simulink model "sampleModel7293_pp_1_1_mu"  (R2018a)
settings: Solver=VariableStepAuto  StartTime=0.0  StopTime=10.0  RelTol=1e-3
undefined symbols (not defined in the file): DiscIntNeverNeededParam
libraries: simulink x367
(part 10 of 13)

== system sampleModel7293_pp_1_1_mu/cfblk199/cfblk13 ==
  cfblk1 : Inport
  cfblk5 : Inport  Port=2
  cfblk6 : Inport  Port=3
  Action Port : ActionPort  ActionType=else
  cfblk3 : DiscreteFilter
  cfblk4 : simulink/Continuous/PID Controller  Controller=PID  TimeDomain=Discrete-time  SampleTime=-1  IntegratorMethod=Forward Euler  FilterMethod=Forward Euler  Form=Parallel  UseFilter=on  ControllerParametersSource=internal  P=1  I=1  D=0  N=100  InitialConditionSource=internal  InitialConditionForIntegrator=0  InitialConditionForFilter=0  ExternalReset=none  LimitOutput=off  UpperSaturationLimit=inf  LowerSaturationLimit=-inf  LinearizeAsGain=off  AntiWindupMode=none  Kb=1  TrackingMode=off  Kt=1  PParamMin=[]  PParamMax=[]  IParamMin=[]  IParamMax=[]  DParamMin=[]  DParamMax=[]  NParamMin=[]  NParamMax=[]  KbParamMin=[]  KbParamMax=[]  KtParamMin=[]  KtParamMax=[]  POutMin=[]  POutMax=[]  IOutMin=[]  IOutMax=[]  DOutMin=[]  DOutMax=[]  NOutMin=[]  NOutMax=[]  KbOutMin=[]  KbOutMax=[]  KtOutMin=[]  KtOutMax=[]  IntegratorOutMin=[]  IntegratorOutMax=[]  FilterOutMin=[]  FilterOutMax=[]  SumOutMin=[]  SumOutMax=[]  SumI1OutMin=[]  SumI1OutMax=[]  SumI2OutMin=[]  SumI2OutMax=[]  SumI3OutMin=[]  SumI3OutMax=[]  SumDOutMin=[]  SumDOutMax=[]  SaturationOutMin=[]  SaturationOutMax=[]  IntegratorContinuousStateAttributes=''  IntegratorStateMustResolveToSignalObject=off  IntegratorRTWStateStorageClass=Auto  FilterContinuousStateAttributes=''  FilterStateMustResolveToSignalObject=off  FilterRTWStateStorageClass=Auto  DifferentiatorICPrevScaledInput=0  DifferentiatorOutMin=[]  DifferentiatorOutMax=[]  FilterDiffOutCoefMin=[]  FilterDiffOutCoefMax=[]  SumDenOutMin=[]  SumDenOutMax=[]  SumNumOutMin=[]  SumNumOutMax=[]  ReciprocalOutMin=[]  ReciprocalOutMax=[]  DivideOutMin=[]  DivideOutMax=[]  TunerSelectOption=Transfer Function Based (PID Tuner App)
  cyemi_1105 : DataTypeConversion  OutDataTypeStr=double
  cyemi_1106 : DataTypeConversion  OutDataTypeStr=double
  cfblk2 : Outport
  cfblk7 : Outport  Port=2
  cfblk8 : Outport  Port=3
  cfblk9 : Outport  Port=4
  cfblk10 : Outport  Port=5
  wires:
  cfblk5/1 -> cfblk2/1, cfblk9/1
  cfblk6/1 -> cfblk10/1, cyemi_1106/1
  cfblk3/1 -> cfblk8/1
  cfblk4/1 -> cfblk7/1
  cyemi_1105/1 -> cfblk3/1
  cfblk1/1 -> cyemi_1105/1
  cyemi_1106/1 -> cfblk4/1

== system sampleModel7293_pp_1_1_mu/cfblk199/cfblk14 ==
  cfblk1 : Inport
  cfblk5 : Inport  Port=2
  cfblk6 : Inport  Port=3
  Action Port : ActionPort  ActionType=then
  cfblk3 : simulink/Discrete/Transfer Fcn First Order  PoleZ=0.95  ICPrevOutput=0.0  DoSatur=off
      settings: SourceProductName=Simulink
  cfblk4 : DiscreteZeroPole  Poles=[0 0.5]  Gain=1  SampleTime=-1
  cyemi_1110 : DataTypeConversion  OutDataTypeStr=double
  cyemi_1111 : DataTypeConversion  OutDataTypeStr=double
  cfblk2 : Outport
  cfblk7 : Outport  Port=2
  wires:
  cfblk6/1 -> cfblk7/1
  cfblk3/1 -> cfblk2/1
  cyemi_1110/1 -> cfblk3/1
  cfblk1/1 -> cyemi_1110/1
  cyemi_1111/1 -> cfblk4/1
  cfblk5/1 -> cyemi_1111/1

== system sampleModel7293_pp_1_1_mu/cfblk199/cfblk15 ==
  cfblk1 : Inport
  cfblk9 : Inport  Port=2
  cfblk10 : Inport  Port=3
  cfblk11 : Inport  Port=4
  Action Port : ActionPort  ActionType=else
  cfblk3 : DiscreteIntegrator  SampleTime=-1  OutDataTypeStr=double  ICPrevOutput=DiscIntNeverNeededParam  ICPrevScaledInput=DiscIntNeverNeededParam
  cfblk4 : simulink/Continuous/PID Controller (2DOF)  Controller=PID  TimeDomain=Discrete-time  SampleTime=-1  IntegratorMethod=Forward Euler  FilterMethod=Forward Euler  Form=Parallel  UseFilter=on  ControllerParametersSource=internal  P=1  I=1  D=0  N=100  b=1  c=1  InitialConditionSource=internal  InitialConditionForIntegrator=0  InitialConditionForFilter=0  ExternalReset=none  LimitOutput=off  UpperSaturationLimit=inf  LowerSaturationLimit=-inf  LinearizeAsGain=off  AntiWindupMode=none  Kb=1  TrackingMode=off  Kt=1  PParamMin=[]  PParamMax=[]  IParamMin=[]  IParamMax=[]  DParamMin=[]  DParamMax=[]  NParamMin=[]  NParamMax=[]  bParamMin=[]  bParamMax=[]  cParamMin=[]  cParamMax=[]  KbParamMin=[]  KbParamMax=[]  KtParamMin=[]  KtParamMax=[]  POutMin=[]  POutMax=[]  IOutMin=[]  IOutMax=[]  DOutMin=[]  DOutMax=[]  NOutMin=[]  NOutMax=[]  bOutMin=[]  bOutMax=[]  cOutMin=[]  cOutMax=[]  KbOutMin=[]  KbOutMax=[]  KtOutMin=[]  KtOutMax=[]  IntegratorOutMin=[]  IntegratorOutMax=[]  FilterOutMin=[]  FilterOutMax=[]  SumOutMin=[]  SumOutMax=[]  Sum1OutMin=[]  Sum1OutMax=[]  Sum2OutMin=[]  Sum2OutMax=[]  Sum3OutMin=[]  Sum3OutMax=[]  SumI1OutMin=[]  SumI1OutMax=[]  SumI2OutMin=[]  SumI2OutMax=[]  SumI3OutMin=[]  SumI3OutMax=[]  SumDOutMin=[]  SumDOutMax=[]  SaturationOutMin=[]  SaturationOutMax=[]  IntegratorContinuousStateAttributes=''  IntegratorStateMustResolveToSignalObject=off  IntegratorRTWStateStorageClass=Auto  FilterContinuousStateAttributes=''  FilterStateMustResolveToSignalObject=off  FilterRTWStateStorageClass=Auto  DifferentiatorICPrevScaledInput=0  DifferentiatorOutMin=[]  DifferentiatorOutMax=[]  FilterDiffOutCoefMin=[]  FilterDiffOutCoefMax=[]  SumDenOutMin=[]  SumDenOutMax=[]  SumNumOutMin=[]  SumNumOutMax=[]  ReciprocalOutMin=[]  ReciprocalOutMax=[]  DivideOutMin=[]  DivideOutMax=[]  TunerSelectOption=Transfer Function Based (PID Tuner App)
  cfblk5 : simulink/Discrete/Transfer Fcn Real Zero  ZeroZ=0.75  ICPrevInput=0.0  DoSatur=off
      settings: SourceProductName=Simulink  SourceProductBaseCode=SL
  cfblk6 : DiscreteFilter
  cfblk7 : simulink/Continuous/PID Controller  Controller=PID  TimeDomain=Discrete-time  SampleTime=-1  IntegratorMethod=Forward Euler  FilterMethod=Forward Euler  Form=Parallel  UseFilter=on  ControllerParametersSource=internal  P=1  I=1  D=0  N=100  InitialConditionSource=internal  InitialConditionForIntegrator=0  InitialConditionForFilter=0  ExternalReset=none  LimitOutput=off  UpperSaturationLimit=inf  LowerSaturationLimit=-inf  LinearizeAsGain=off  AntiWindupMode=none  Kb=1  TrackingMode=off  Kt=1  PParamMin=[]  PParamMax=[]  IParamMin=[]  IParamMax=[]  DParamMin=[]  DParamMax=[]  NParamMin=[]  NParamMax=[]  KbParamMin=[]  KbParamMax=[]  KtParamMin=[]  KtParamMax=[]  POutMin=[]  POutMax=[]  IOutMin=[]  IOutMax=[]  DOutMin=[]  DOutMax=[]  NOutMin=[]  NOutMax=[]  KbOutMin=[]  KbOutMax=[]  KtOutMin=[]  KtOutMax=[]  IntegratorOutMin=[]  IntegratorOutMax=[]  FilterOutMin=[]  FilterOutMax=[]  SumOutMin=[]  SumOutMax=[]  SumI1OutMin=[]  SumI1OutMax=[]  SumI2OutMin=[]  SumI2OutMax=[]  SumI3OutMin=[]  SumI3OutMax=[]  SumDOutMin=[]  SumDOutMax=[]  SaturationOutMin=[]  SaturationOutMax=[]  IntegratorContinuousStateAttributes=''  IntegratorStateMustResolveToSignalObject=off  IntegratorRTWStateStorageClass=Auto  FilterContinuousStateAttributes=''  FilterStateMustResolveToSignalObject=off  FilterRTWStateStorageClass=Auto  DifferentiatorICPrevScaledInput=0  DifferentiatorOutMin=[]  DifferentiatorOutMax=[]  FilterDiffOutCoefMin=[]  FilterDiffOutCoefMax=[]  SumDenOutMin=[]  SumDenOutMax=[]  SumNumOutMin=[]  SumNumOutMax=[]  ReciprocalOutMin=[]  ReciprocalOutMax=[]  DivideOutMin=[]  DivideOutMax=[]  TunerSelectOption=Transfer Function Based (PID Tuner App)
  cfblk8 : simulink/Discrete/Difference  ICPrevInput=0.0  OutMin=[]  OutMax=[]  OutDataTypeStr=double  OutputDataTypeScalingMode=double  OutDataType=fixdt(1, 16)  OutScaling=2^-10  DoSatur=off
  cyemi_{1116..1122} (7 alike) : DataTypeConversion  OutDataTypeStr=double
  cfblk2 : Outport
  cfblk12 : Outport  Port=2
  cfblk13 : Outport  Port=3
  cfblk14 : Outport  Port=4
  wires:
  cfblk4/1 -> cfblk12/1
  cfblk11/1 -> cyemi_1117/1, cyemi_1120/1
  cfblk8/1 -> cfblk14/1
  cfblk6/1 -> cfblk2/1
  cfblk1/1 -> cfblk13/1
  cyemi_1116/1 -> cfblk3/1
  cfblk7/1 -> cyemi_1116/1
  cyemi_1117/1 -> cfblk4/1
  cyemi_1118/1 -> cfblk4/2
  cfblk10/1 -> cyemi_1118/1
  cyemi_1119/1 -> cfblk5/1
  cfblk9/1 -> cyemi_1119/1
  cyemi_1120/1 -> cfblk6/1
  cyemi_1121/1 -> cfblk7/1
  cfblk5/1 -> cyemi_1121/1
  cyemi_1122/1 -> cfblk8/1
  cfblk3/1 -> cyemi_1122/1

== system sampleModel7293_pp_1_1_mu/cfblk199/cfblk22 ==
  emi_1180 : Inport
  Action Port : ActionPort  ActionType=then
  cfblk22 : Delay
  emi_1181 : Outport
  wires:
  emi_1180/1 -> cfblk22/1
  cfblk22/1 -> emi_1181/1

== system sampleModel7293_pp_1_1_mu/cfblk199/cfblk24 ==
  emi_1807 : Inport
  Action Port : ActionPort  ActionType=then
  cfblk24 : Delay
  emi_1808 : Outport
  wires:
  emi_1807/1 -> cfblk24/1
  cfblk24/1 -> emi_1808/1

== system sampleModel7293_pp_1_1_mu/cfblk199/cfblk5 ==
  emi_1529 : Inport
  Action Port : ActionPort  ActionType=then
  cfblk5 : DiscreteFir
  emi_1530 : Outport
  wires:
  emi_1529/1 -> cfblk5/1
  cfblk5/1 -> emi_1530/1

== system sampleModel7293_pp_1_1_mu/cfblk199/cfblk7 ==
  emi_832 : Inport
  Action Port : ActionPort  ActionType=then
  cfblk7 : UnitDelay  SampleTime=-1
  emi_833 : Outport
  wires:
  emi_832/1 -> cfblk7/1
  cfblk7/1 -> emi_833/1

== system sampleModel7293_pp_1_1_mu/cfblk199/emi_1182 ==
  Action Port : ActionPort  ActionType=else
  emi_1183 : Assertion

== system sampleModel7293_pp_1_1_mu/cfblk199/emi_1531 ==
  Action Port : ActionPort  ActionType=else
  emi_1532 : Assertion

== system sampleModel7293_pp_1_1_mu/cfblk199/emi_1809 ==
  Action Port : ActionPort  ActionType=else
  emi_1810 : Assertion

== system sampleModel7293_pp_1_1_mu/cfblk199/emi_834 ==
  Action Port : ActionPort  ActionType=else
  emi_835 : Assertion

== system sampleModel7293_pp_1_1_mu/cfblk200/cfblk11 ==
  cfblk1 : Inport
  Action Port : ActionPort  ActionType=then
  cfblk10 : simulink/Discrete/Transfer Fcn Lead or Lag  PoleZ=0.95  ZeroZ=0.75  ICPrevOutput=0.0  ICPrevInput=0.0  DoSatur=off
      settings: SourceProductName=Simulink  SourceProductBaseCode=SL
  cfblk11 : simulink/Discrete/Tapped Delay  vinit=0.0  samptime=-1  NumDelays=1  DelayOrder=Oldest  includeCurrent=off
  cfblk12 : Delay
  cfblk3 : Subsystem  TreatAsAtomicUnit=on
  cfblk4 : DiscreteTransferFcn
  cfblk5 : simulink/Continuous/PID Controller  Controller=PID  TimeDomain=Discrete-time  SampleTime=-1  IntegratorMethod=Forward Euler  FilterMethod=Forward Euler  Form=Parallel  UseFilter=on  ControllerParametersSource=internal  P=1  I=1  D=0  N=100  InitialConditionSource=internal  InitialConditionForIntegrator=0  InitialConditionForFilter=0  ExternalReset=none  LimitOutput=off  UpperSaturationLimit=inf  LowerSaturationLimit=-inf  LinearizeAsGain=off  AntiWindupMode=none  Kb=1  TrackingMode=off  Kt=1  PParamMin=[]  PParamMax=[]  IParamMin=[]  IParamMax=[]  DParamMin=[]  DParamMax=[]  NParamMin=[]  NParamMax=[]  KbParamMin=[]  KbParamMax=[]  KtParamMin=[]  KtParamMax=[]  POutMin=[]  POutMax=[]  IOutMin=[]  IOutMax=[]  DOutMin=[]  DOutMax=[]  NOutMin=[]  NOutMax=[]  KbOutMin=[]  KbOutMax=[]  KtOutMin=[]  KtOutMax=[]  IntegratorOutMin=[]  IntegratorOutMax=[]  FilterOutMin=[]  FilterOutMax=[]  SumOutMin=[]  SumOutMax=[]  SumI1OutMin=[]  SumI1OutMax=[]  SumI2OutMin=[]  SumI2OutMax=[]  SumI3OutMin=[]  SumI3OutMax=[]  SumDOutMin=[]  SumDOutMax=[]  SaturationOutMin=[]  SaturationOutMax=[]  IntegratorContinuousStateAttributes=''  IntegratorStateMustResolveToSignalObject=off  IntegratorRTWStateStorageClass=Auto  FilterContinuousStateAttributes=''  FilterStateMustResolveToSignalObject=off  FilterRTWStateStorageClass=Auto  DifferentiatorICPrevScaledInput=0  DifferentiatorOutMin=[]  DifferentiatorOutMax=[]  FilterDiffOutCoefMin=[]  FilterDiffOutCoefMax=[]  SumDenOutMin=[]  SumDenOutMax=[]  SumNumOutMin=[]  SumNumOutMax=[]  ReciprocalOutMin=[]  ReciprocalOutMax=[]  DivideOutMin=[]  DivideOutMax=[]  TunerSelectOption=Transfer Function Based (PID Tuner App)
  cfblk6 : DiscreteZeroPole  Poles=[0 0.5]  Gain=1  SampleTime=-1
  cfblk7 : Subsystem  TreatAsAtomicUnit=on
  cfblk8 : simulink/Discrete/Transfer Fcn First Order  PoleZ=0.95  ICPrevOutput=0.0  DoSatur=off
      settings: SourceProductName=Simulink
  cfblk9 : simulink/Discrete/Transfer Fcn Real Zero  ZeroZ=0.75  ICPrevInput=0.0  DoSatur=off
      settings: SourceProductName=Simulink  SourceProductBaseCode=SL
  cyemi_{1147..1156} (10 alike) : DataTypeConversion  OutDataTypeStr=double
  emi_968 : Subsystem  TreatAsAtomicUnit=on
  emi_970 : If  IfExpression=Inf <= u1
  emi_971 : DataTypeConversion  OutDataTypeStr=double
  emi_996 : Subsystem  TreatAsAtomicUnit=on
  emi_998 : If  IfExpression=Inf <= u1
  emi_999 : DataTypeConversion  OutDataTypeStr=double
  cfblk2 : Outport
  wires:
  cfblk11/1 -> cfblk2/1
  cyemi_1147/1 -> cfblk10/1
  cfblk8/1 -> cyemi_1147/1
  cyemi_1148/1 -> cfblk11/1
  cfblk5/1 -> cyemi_1148/1
  cyemi_1149/1 -> cfblk12/1
  cfblk10/1 -> cyemi_1149/1
  cfblk9/1 -> cyemi_1150/1
  cyemi_1151/1 -> cfblk4/1
  cyemi_1152/1 -> cfblk5/1
  cfblk4/1 -> cyemi_1152/1
  cyemi_1153/1 -> cfblk6/1
  cfblk1/1 -> cyemi_1153/1
  cyemi_1155/1 -> cfblk8/1
  cfblk12/1 -> cyemi_1155/1
  cyemi_1156/1 -> cfblk9/1
  cfblk6/1 -> cyemi_1156/1, emi_999/1
  cyemi_1150/1 -> cfblk3/1(emi_966)
  cfblk3/1(emi_967) -> cyemi_1154/1
  emi_970/1 -> cfblk3/Action
  emi_970/2 -> emi_968/Action
  emi_971/1 -> emi_970/1
  cyemi_1154/1 -> cfblk7/1(emi_994)
  cfblk7/1(emi_995) -> emi_971/1, cyemi_1151/1
  emi_998/1 -> cfblk7/Action
  emi_998/2 -> emi_996/Action
  emi_999/1 -> emi_998/1

== system sampleModel7293_pp_1_1_mu/cfblk200/cfblk12 ==
  cfblk1 : Inport
  cfblk9 : Inport  Port=2
  Action Port : ActionPort  ActionType=else
  cfblk10 : Subsystem  TreatAsAtomicUnit=on
  cfblk11 : Subsystem  TreatAsAtomicUnit=on
  cfblk3 : Subsystem  TreatAsAtomicUnit=on
  cfblk4 : Subsystem  TreatAsAtomicUnit=on
  cfblk5 : DiscreteFir
  cfblk6 : DiscreteTransferFcn
  cfblk7 : simulink/Continuous/PID Controller (2DOF)  Controller=PID  TimeDomain=Discrete-time  SampleTime=-1  IntegratorMethod=Forward Euler  FilterMethod=Forward Euler  Form=Parallel  UseFilter=on  ControllerParametersSource=internal  P=1  I=1  D=0  N=100  b=1  c=1  InitialConditionSource=internal  InitialConditionForIntegrator=0  InitialConditionForFilter=0  ExternalReset=none  LimitOutput=off  UpperSaturationLimit=inf  LowerSaturationLimit=-inf  LinearizeAsGain=off  AntiWindupMode=none  Kb=1  TrackingMode=off  Kt=1  PParamMin=[]  PParamMax=[]  IParamMin=[]  IParamMax=[]  DParamMin=[]  DParamMax=[]  NParamMin=[]  NParamMax=[]  bParamMin=[]  bParamMax=[]  cParamMin=[]  cParamMax=[]  KbParamMin=[]  KbParamMax=[]  KtParamMin=[]  KtParamMax=[]  POutMin=[]  POutMax=[]  IOutMin=[]  IOutMax=[]  DOutMin=[]  DOutMax=[]  NOutMin=[]  NOutMax=[]  bOutMin=[]  bOutMax=[]  cOutMin=[]  cOutMax=[]  KbOutMin=[]  KbOutMax=[]  KtOutMin=[]  KtOutMax=[]  IntegratorOutMin=[]  IntegratorOutMax=[]  FilterOutMin=[]  FilterOutMax=[]  SumOutMin=[]  SumOutMax=[]  Sum1OutMin=[]  Sum1OutMax=[]  Sum2OutMin=[]  Sum2OutMax=[]  Sum3OutMin=[]  Sum3OutMax=[]  SumI1OutMin=[]  SumI1OutMax=[]  SumI2OutMin=[]  SumI2OutMax=[]  SumI3OutMin=[]  SumI3OutMax=[]  SumDOutMin=[]  SumDOutMax=[]  SaturationOutMin=[]  SaturationOutMax=[]  IntegratorContinuousStateAttributes=''  IntegratorStateMustResolveToSignalObject=off  IntegratorRTWStateStorageClass=Auto  FilterContinuousStateAttributes=''  FilterStateMustResolveToSignalObject=off  FilterRTWStateStorageClass=Auto  DifferentiatorICPrevScaledInput=0  DifferentiatorOutMin=[]  DifferentiatorOutMax=[]  FilterDiffOutCoefMin=[]  FilterDiffOutCoefMax=[]  SumDenOutMin=[]  SumDenOutMax=[]  SumNumOutMin=[]  SumNumOutMax=[]  ReciprocalOutMin=[]  ReciprocalOutMax=[]  DivideOutMin=[]  DivideOutMax=[]  TunerSelectOption=Transfer Function Based (PID Tuner App)
  cfblk8 : UnitDelay  SampleTime=-1
  cyemi_{1159..1168} (10 alike) : DataTypeConversion  OutDataTypeStr=double
  emi_1116 : Subsystem  TreatAsAtomicUnit=on
  emi_{291,865,1118,1277} (4 alike) : If  IfExpression=Inf <= u1
  emi_{292,866,1119,1278} (4 alike) : DataTypeConversion  OutDataTypeStr=double
  emi_1275 : Subsystem  TreatAsAtomicUnit=on
  emi_289 : Subsystem  TreatAsAtomicUnit=on
  emi_863 : Subsystem  TreatAsAtomicUnit=on
  cfblk2 : Outport
  wires:
  cfblk5/1 -> cfblk2/1
  cfblk6/1 -> cyemi_1160/1, cyemi_1161/1
  cfblk1/1 -> cyemi_1162/1
  cyemi_1164/1 -> cfblk5/1
  cfblk8/1 -> cyemi_1164/1, emi_292/1, emi_1278/1
  cyemi_1165/1 -> cfblk6/1
  cfblk7/1 -> cyemi_1165/1
  cyemi_1166/1 -> cfblk7/1
  cyemi_1167/1 -> cfblk7/2
  cyemi_1168/1 -> cfblk8/1
  cfblk9/1 -> cyemi_1168/1
  cyemi_1162/1 -> cfblk4/1(emi_286)
  cyemi_1163/1 -> cfblk4/2(emi_287)
  cfblk4/1(emi_288) -> cyemi_1167/1
  emi_291/1 -> cfblk4/Action
  emi_291/2 -> emi_289/Action
  emi_292/1 -> emi_291/1
  cyemi_1161/1 -> cfblk3/1(emi_861)
  cfblk3/1(emi_862) -> cyemi_1159/1
  emi_865/1 -> cfblk3/Action
  emi_865/2 -> emi_863/Action
  emi_866/1 -> emi_865/1
  cyemi_1160/1 -> cfblk11/1(emi_1114)
  cfblk11/1(emi_1115) -> emi_866/1, cyemi_1163/1
  emi_1118/1 -> cfblk11/Action
  emi_1118/2 -> emi_1116/Action
  emi_1119/1 -> emi_1118/1
  cyemi_1159/1 -> cfblk10/1(emi_1273)
  cfblk10/1(emi_1274) -> emi_1119/1, cyemi_1166/1
  emi_1277/1 -> cfblk10/Action
  emi_1277/2 -> emi_1275/Action
  emi_1278/1 -> emi_1277/1

== system sampleModel7293_pp_1_1_mu/cfblk200/cfblk3 ==
  emi_924 : Inport
  Action Port : ActionPort  ActionType=then
  cfblk3 : simulink/Discrete/Tapped Delay  vinit=0.0  samptime=-1  NumDelays=1  DelayOrder=Oldest  includeCurrent=off
  emi_925 : Outport
  wires:
  emi_924/1 -> cfblk3/1
  cfblk3/1 -> emi_925/1

== system sampleModel7293_pp_1_1_mu/cfblk200/cfblk4 ==
  emi_639 : Inport
  Action Port : ActionPort  ActionType=then
  cfblk4 : simulink/Discrete/Difference  ICPrevInput=0.0  OutMin=[]  OutMax=[]  OutDataTypeStr=double  OutputDataTypeScalingMode=double  OutDataType=fixdt(1, 16)  OutScaling=2^-10  DoSatur=off
  emi_640 : Outport
  wires:
  emi_639/1 -> cfblk4/1
  cfblk4/1 -> emi_640/1

== system sampleModel7293_pp_1_1_mu/cfblk200/emi_641 ==
  Action Port : ActionPort  ActionType=else
  emi_642 : Assertion

== system sampleModel7293_pp_1_1_mu/cfblk200/emi_926 ==
  Action Port : ActionPort  ActionType=else
  emi_927 : Assertion

== system sampleModel7293_pp_1_1_mu/cfblk201/cfblk12 ==
  emi_1259 : Inport
  Action Port : ActionPort  ActionType=then
  cfblk12 : DiscreteTransferFcn
  emi_1260 : Outport
  wires:
  emi_1259/1 -> cfblk12/1
  cfblk12/1 -> emi_1260/1

== system sampleModel7293_pp_1_1_mu/cfblk201/cfblk4 ==
  emi_472 : Inport
  emi_473 : Inport  Port=2
  Action Port : ActionPort  ActionType=then
  cfblk4 : Delay  DelayLengthSource=Input port
      settings: InputPortMap=u0,p1
  emi_474 : Outport
  wires:
  emi_472/1 -> cfblk4/1
  emi_473/1 -> cfblk4/2
  cfblk4/1 -> emi_474/1

== system sampleModel7293_pp_1_1_mu/cfblk201/cfblk7 ==
  emi_910 : Inport
  Action Port : ActionPort  ActionType=then
  cfblk7 : DiscreteIntegrator  SampleTime=-1  OutDataTypeStr=double  ICPrevOutput=DiscIntNeverNeededParam  ICPrevScaledInput=DiscIntNeverNeededParam
  emi_911 : Outport
  wires:
  emi_910/1 -> cfblk7/1
  cfblk7/1 -> emi_911/1

== system sampleModel7293_pp_1_1_mu/cfblk201/cfblk8 ==
  emi_1308 : Inport
  Action Port : ActionPort  ActionType=then
  cfblk8 : DiscreteStateSpace  SampleTime=-1
  emi_1309 : Outport
  wires:
  emi_1308/1 -> cfblk8/1
  cfblk8/1 -> emi_1309/1

== system sampleModel7293_pp_1_1_mu/cfblk201/emi_1261 ==
  Action Port : ActionPort  ActionType=else
  emi_1262 : Assertion

== system sampleModel7293_pp_1_1_mu/cfblk201/emi_1310 ==
  Action Port : ActionPort  ActionType=else
  emi_1311 : Assertion

== system sampleModel7293_pp_1_1_mu/cfblk201/emi_475 ==
  Action Port : ActionPort  ActionType=else
  emi_476 : Assertion

== system sampleModel7293_pp_1_1_mu/cfblk201/emi_912 ==
  Action Port : ActionPort  ActionType=else
  emi_913 : Assertion

== system sampleModel7293_pp_1_1_mu/cfblk202/cfblk10 ==
  emi_1735 : Inport
  Action Port : ActionPort  ActionType=then
  cfblk10 : DiscreteStateSpace  SampleTime=-1
  emi_1736 : Outport
  wires:
  emi_1735/1 -> cfblk10/1
  cfblk10/1 -> emi_1736/1

== system sampleModel7293_pp_1_1_mu/cfblk202/cfblk13 ==
  emi_1522 : Inport
  Action Port : ActionPort  ActionType=then
  cfblk13 : Delay
  emi_1523 : Outport
  wires:
  emi_1522/1 -> cfblk13/1
  cfblk13/1 -> emi_1523/1

== system sampleModel7293_pp_1_1_mu/cfblk202/cfblk3 ==
  emi_959 : Inport
  Action Port : ActionPort  ActionType=then
  cfblk3 : simulink/Discrete/Tapped Delay  vinit=0.0  samptime=-1  NumDelays=1  DelayOrder=Oldest  includeCurrent=off
  emi_960 : Outport
  wires:
  emi_959/1 -> cfblk3/1
  cfblk3/1 -> emi_960/1

== system sampleModel7293_pp_1_1_mu/cfblk202/cfblk4 ==
  emi_581 : Inport
  Action Port : ActionPort  ActionType=then
  cfblk4 : simulink/Discrete/Transfer Fcn Lead or Lag  PoleZ=0.95  ZeroZ=0.75  ICPrevOutput=0.0  ICPrevInput=0.0  DoSatur=off
      settings: SourceProductName=Simulink  SourceProductBaseCode=SL
  emi_582 : Outport
  wires:
  emi_581/1 -> cfblk4/1
  cfblk4/1 -> emi_582/1

== system sampleModel7293_pp_1_1_mu/cfblk202/cfblk7 ==
  emi_1165 : Inport
  Action Port : ActionPort  ActionType=then
  cfblk7 : DiscreteFir
  emi_1166 : Outport
  wires:
  emi_1165/1 -> cfblk7/1
  cfblk7/1 -> emi_1166/1

== system sampleModel7293_pp_1_1_mu/cfblk202/emi_1167 ==
  Action Port : ActionPort  ActionType=else
  emi_1168 : Assertion

== system sampleModel7293_pp_1_1_mu/cfblk202/emi_1524 ==
  Action Port : ActionPort  ActionType=else
  emi_1525 : Assertion

== system sampleModel7293_pp_1_1_mu/cfblk202/emi_1737 ==
  Action Port : ActionPort  ActionType=else
  emi_1738 : Assertion

== system sampleModel7293_pp_1_1_mu/cfblk202/emi_583 ==
  Action Port : ActionPort  ActionType=else
  emi_584 : Assertion

== system sampleModel7293_pp_1_1_mu/cfblk202/emi_961 ==
  Action Port : ActionPort  ActionType=else
  emi_962 : Assertion

== system sampleModel7293_pp_1_1_mu/cfblk203/cfblk12 ==
  cfblk1 : Inport
  Action Port : ActionPort  ActionType=then
  cfblk10 : Subsystem  TreatAsAtomicUnit=on
  cfblk11 : Delay
  cfblk3 : Subsystem  TreatAsAtomicUnit=on
  cfblk4 : Subsystem  TreatAsAtomicUnit=on
  cfblk5 : Subsystem  TreatAsAtomicUnit=on
  cfblk6 : DiscreteFilter
  cfblk7 : simulink/Discrete/Transfer Fcn Real Zero  ZeroZ=0.75  ICPrevInput=0.0  DoSatur=off
      settings: SourceProductName=Simulink  SourceProductBaseCode=SL
  cfblk8 : simulink/Discrete/Difference  ICPrevInput=0.0  OutMin=[]  OutMax=[]  OutDataTypeStr=double  OutputDataTypeScalingMode=double  OutDataType=fixdt(1, 16)  OutScaling=2^-10  DoSatur=off
  cfblk9 : Subsystem  TreatAsAtomicUnit=on
  cyemi_{1214..1223} (10 alike) : DataTypeConversion  OutDataTypeStr=double
  emi_1197 : Subsystem  TreatAsAtomicUnit=on
  emi_{305,792,1199,1270,1576} (5 alike) : If  IfExpression=Inf <= u1
  emi_{306,793,1200,1271,1577} (5 alike) : DataTypeConversion  OutDataTypeStr=double
  emi_1268 : Subsystem  TreatAsAtomicUnit=on
  emi_1574 : Subsystem  TreatAsAtomicUnit=on
  emi_303 : Subsystem  TreatAsAtomicUnit=on
  emi_790 : Subsystem  TreatAsAtomicUnit=on
  cfblk2 : Outport
  wires:
  cfblk7/1 -> cfblk2/1, cyemi_1217/1
  cyemi_1215/1 -> cfblk11/1
  cfblk8/1 -> cyemi_1215/1
  cfblk11/1 -> cyemi_1218/1
  cyemi_1219/1 -> cfblk6/1
  cfblk1/1 -> cyemi_1219/1
  cyemi_1220/1 -> cfblk7/1
  cfblk6/1 -> cyemi_1220/1
  cyemi_1221/1 -> cfblk8/1
  cyemi_1218/1 -> cfblk5/1(emi_301)
  cfblk5/1(emi_302) -> cyemi_1221/1
  emi_305/1 -> cfblk5/Action
  emi_305/2 -> emi_303/Action
  emi_306/1 -> emi_305/1
  cyemi_1216/1 -> cfblk3/1(emi_788)
  cfblk3/1(emi_789) -> cyemi_1214/1
  emi_792/1 -> cfblk3/Action
  emi_792/2 -> emi_790/Action
  emi_793/1 -> emi_792/1
  cyemi_1217/1 -> cfblk4/1(emi_1195)
  cfblk4/1(emi_1196) -> emi_793/1, cyemi_1223/1, emi_1577/1
  emi_1199/1 -> cfblk4/Action
  emi_1199/2 -> emi_1197/Action
  emi_1200/1 -> emi_1199/1
  cyemi_1214/1 -> cfblk10/1(emi_1266)
  cfblk10/1(emi_1267) -> emi_306/1, cyemi_1222/1
  emi_1270/1 -> cfblk10/Action
  emi_1270/2 -> emi_1268/Action
  emi_1271/1 -> emi_1270/1
  cyemi_1222/1 -> cfblk9/1(emi_1571)
  cyemi_1223/1 -> cfblk9/2(emi_1572)
  cfblk9/1(emi_1573) -> emi_1271/1, emi_1200/1, cyemi_1216/1
  emi_1576/1 -> cfblk9/Action
  emi_1576/2 -> emi_1574/Action
  emi_1577/1 -> emi_1576/1

== system sampleModel7293_pp_1_1_mu/cfblk203/cfblk13 ==
  cfblk1 : Inport
  cfblk12 : Inport  Port=2
  cfblk13 : Inport  Port=3
  Action Port : ActionPort  ActionType=else
  cfblk10 : simulink/Continuous/PID Controller  Controller=PID  TimeDomain=Discrete-time  SampleTime=-1  IntegratorMethod=Forward Euler  FilterMethod=Forward Euler  Form=Parallel  UseFilter=on  ControllerParametersSource=internal  P=1  I=1  D=0  N=100  InitialConditionSource=internal  InitialConditionForIntegrator=0  InitialConditionForFilter=0  ExternalReset=none  LimitOutput=off  UpperSaturationLimit=inf  LowerSaturationLimit=-inf  LinearizeAsGain=off  AntiWindupMode=none  Kb=1  TrackingMode=off  Kt=1  PParamMin=[]  PParamMax=[]  IParamMin=[]  IParamMax=[]  DParamMin=[]  DParamMax=[]  NParamMin=[]  NParamMax=[]  KbParamMin=[]  KbParamMax=[]  KtParamMin=[]  KtParamMax=[]  POutMin=[]  POutMax=[]  IOutMin=[]  IOutMax=[]  DOutMin=[]  DOutMax=[]  NOutMin=[]  NOutMax=[]  KbOutMin=[]  KbOutMax=[]  KtOutMin=[]  KtOutMax=[]  IntegratorOutMin=[]  IntegratorOutMax=[]  FilterOutMin=[]  FilterOutMax=[]  SumOutMin=[]  SumOutMax=[]  SumI1OutMin=[]  SumI1OutMax=[]  SumI2OutMin=[]  SumI2OutMax=[]  SumI3OutMin=[]  SumI3OutMax=[]  SumDOutMin=[]  SumDOutMax=[]  SaturationOutMin=[]  SaturationOutMax=[]  IntegratorContinuousStateAttributes=''  IntegratorStateMustResolveToSignalObject=off  IntegratorRTWStateStorageClass=Auto  FilterContinuousStateAttributes=''  FilterStateMustResolveToSignalObject=off  FilterRTWStateStorageClass=Auto  DifferentiatorICPrevScaledInput=0  DifferentiatorOutMin=[]  DifferentiatorOutMax=[]  FilterDiffOutCoefMin=[]  FilterDiffOutCoefMax=[]  SumDenOutMin=[]  SumDenOutMax=[]  SumNumOutMin=[]  SumNumOutMax=[]  ReciprocalOutMin=[]  ReciprocalOutMax=[]  DivideOutMin=[]  DivideOutMax=[]  TunerSelectOption=Transfer Function Based (PID Tuner App)
  cfblk11 : Subsystem  TreatAsAtomicUnit=on
  cfblk3 : Subsystem  TreatAsAtomicUnit=on
  cfblk4 : Subsystem  TreatAsAtomicUnit=on
  cfblk5 : DiscreteZeroPole  Poles=[0 0.5]  Gain=1  SampleTime=-1
  cfblk6 : simulink/Discrete/Transfer Fcn Real Zero  ZeroZ=0.75  ICPrevInput=0.0  DoSatur=off
      settings: SourceProductName=Simulink  SourceProductBaseCode=SL
  cfblk7 : DiscreteTransferFcn
  cfblk8 : DiscreteFir
  cfblk9 : simulink/Continuous/PID Controller (2DOF)  Controller=PID  TimeDomain=Discrete-time  SampleTime=-1  IntegratorMethod=Forward Euler  FilterMethod=Forward Euler  Form=Parallel  UseFilter=on  ControllerParametersSource=internal  P=1  I=1  D=0  N=100  b=1  c=1  InitialConditionSource=internal  InitialConditionForIntegrator=0  InitialConditionForFilter=0  ExternalReset=none  LimitOutput=off  UpperSaturationLimit=inf  LowerSaturationLimit=-inf  LinearizeAsGain=off  AntiWindupMode=none  Kb=1  TrackingMode=off  Kt=1  PParamMin=[]  PParamMax=[]  IParamMin=[]  IParamMax=[]  DParamMin=[]  DParamMax=[]  NParamMin=[]  NParamMax=[]  bParamMin=[]  bParamMax=[]  cParamMin=[]  cParamMax=[]  KbParamMin=[]  KbParamMax=[]  KtParamMin=[]  KtParamMax=[]  POutMin=[]  POutMax=[]  IOutMin=[]  IOutMax=[]  DOutMin=[]  DOutMax=[]  NOutMin=[]  NOutMax=[]  bOutMin=[]  bOutMax=[]  cOutMin=[]  cOutMax=[]  KbOutMin=[]  KbOutMax=[]  KtOutMin=[]  KtOutMax=[]  IntegratorOutMin=[]  IntegratorOutMax=[]  FilterOutMin=[]  FilterOutMax=[]  SumOutMin=[]  SumOutMax=[]  Sum1OutMin=[]  Sum1OutMax=[]  Sum2OutMin=[]  Sum2OutMax=[]  Sum3OutMin=[]  Sum3OutMax=[]  SumI1OutMin=[]  SumI1OutMax=[]  SumI2OutMin=[]  SumI2OutMax=[]  SumI3OutMin=[]  SumI3OutMax=[]  SumDOutMin=[]  SumDOutMax=[]  SaturationOutMin=[]  SaturationOutMax=[]  IntegratorContinuousStateAttributes=''  IntegratorStateMustResolveToSignalObject=off  IntegratorRTWStateStorageClass=Auto  FilterContinuousStateAttributes=''  FilterStateMustResolveToSignalObject=off  FilterRTWStateStorageClass=Auto  DifferentiatorICPrevScaledInput=0  DifferentiatorOutMin=[]  DifferentiatorOutMax=[]  FilterDiffOutCoefMin=[]  FilterDiffOutCoefMax=[]  SumDenOutMin=[]  SumDenOutMax=[]  SumNumOutMin=[]  SumNumOutMax=[]  ReciprocalOutMin=[]  ReciprocalOutMax=[]  DivideOutMin=[]  DivideOutMax=[]  TunerSelectOption=Transfer Function Based (PID Tuner App)
  cyemi_{1227..1236} (10 alike) : DataTypeConversion  OutDataTypeStr=double
  emi_131 : Subsystem  TreatAsAtomicUnit=on
  emi_133 : If  IfExpression=0 <= u1
  emi_134 : DataTypeConversion  OutDataTypeStr=double
  emi_1950 : Subsystem  TreatAsAtomicUnit=on
  emi_1952 : If  IfExpression=0 <= u1
  emi_1953 : DataTypeConversion  OutDataTypeStr=double
  emi_217 : Subsystem  TreatAsAtomicUnit=on
  emi_219 : If  IfExpression=0 <= u1
  emi_220 : DataTypeConversion  OutDataTypeStr=double
  cfblk2 : Outport
  cfblk14 : Outport  Port=2
  cfblk15 : Outport  Port=3
  wires:
  cfblk6/1 -> cfblk15/1
  cfblk13/1 -> cfblk14/1
  cfblk8/1 -> cfblk2/1, emi_220/1
  cyemi_1227/1 -> cfblk10/1
  cfblk12/1 -> cyemi_1227/1
  cfblk10/1 -> cyemi_1228/1
  cyemi_1231/1 -> cfblk5/1
  cyemi_1232/1 -> cfblk6/1
  cfblk9/1 -> cyemi_1232/1
  cyemi_1233/1 -> cfblk7/1
  cfblk5/1 -> cyemi_1233/1
  cyemi_1234/1 -> cfblk8/1
  cyemi_1235/1 -> cfblk9/1
  cfblk1/1 -> cyemi_1235/1
  cyemi_1236/1 -> cfblk9/2
  cfblk7/1 -> cyemi_1236/1, emi_1953/1
  cyemi_1229/1 -> cfblk3/1(emi_129)
  cfblk3/1(emi_130) -> cyemi_1234/1
  emi_133/1 -> cfblk3/Action
  emi_133/2 -> emi_131/Action
  emi_134/1 -> emi_133/1
  cyemi_1228/1 -> cfblk11/1(emi_215)
  cfblk11/1(emi_216) -> emi_134/1, cyemi_1230/1, cyemi_1229/1
  emi_219/1 -> cfblk11/Action
  emi_219/2 -> emi_217/Action
  emi_220/1 -> emi_219/1
  cyemi_1230/1 -> cfblk4/1(emi_1948)
  cfblk4/1(emi_1949) -> cyemi_1231/1
  emi_1952/1 -> cfblk4/Action
  emi_1952/2 -> emi_1950/Action
  emi_1953/1 -> emi_1952/1

== system sampleModel7293_pp_1_1_mu/cfblk203/cfblk16 ==
  emi_136 : Inport
  Action Port : ActionPort  ActionType=then
  cfblk16 : Delay
  emi_137 : Outport
  wires:
  emi_136/1 -> cfblk16/1
  cfblk16/1 -> emi_137/1

== system sampleModel7293_pp_1_1_mu/cfblk203/cfblk17 ==
  emi_1301 : Inport
  Action Port : ActionPort  ActionType=then
  cfblk17 : Delay
  emi_1302 : Outport
  wires:
  emi_1301/1 -> cfblk17/1
  cfblk17/1 -> emi_1302/1

== system sampleModel7293_pp_1_1_mu/cfblk203/cfblk6 ==
  emi_380 : Inport
  Action Port : ActionPort  ActionType=then
  cfblk6 : Delay
  emi_381 : Outport
  wires:
  emi_380/1 -> cfblk6/1
  cfblk6/1 -> emi_381/1

== system sampleModel7293_pp_1_1_mu/cfblk203/emi_1303 ==
  Action Port : ActionPort  ActionType=else
  emi_1304 : Assertion

== system sampleModel7293_pp_1_1_mu/cfblk203/emi_138 ==
  Action Port : ActionPort  ActionType=else
  emi_139 : Assertion

== system sampleModel7293_pp_1_1_mu/cfblk203/emi_382 ==
  Action Port : ActionPort  ActionType=else
  emi_383 : Assertion

== system sampleModel7293_pp_1_1_mu/cfblk204/cfblk3 ==
  emi_2040 : Inport
  Action Port : ActionPort  ActionType=then
  cfblk3 : simulink/Discrete/Transfer Fcn Real Zero  ZeroZ=0.75  ICPrevInput=0.0  DoSatur=off
      settings: SourceProductName=Simulink  SourceProductBaseCode=SL
  emi_2041 : Outport
  wires:
  emi_2040/1 -> cfblk3/1
  cfblk3/1 -> emi_2041/1

== system sampleModel7293_pp_1_1_mu/cfblk204/cfblk4 ==
  emi_422 : Inport
  Action Port : ActionPort  ActionType=then
  cfblk4 : simulink/Discrete/Transfer Fcn Lead or Lag  PoleZ=0.95  ZeroZ=0.75  ICPrevOutput=0.0  ICPrevInput=0.0  DoSatur=off
      settings: SourceProductName=Simulink  SourceProductBaseCode=SL
  emi_423 : Outport
  wires:
  emi_422/1 -> cfblk4/1
  cfblk4/1 -> emi_423/1

== system sampleModel7293_pp_1_1_mu/cfblk204/emi_2042 ==
  Action Port : ActionPort  ActionType=else
  emi_2043 : Assertion

== system sampleModel7293_pp_1_1_mu/cfblk204/emi_424 ==
  Action Port : ActionPort  ActionType=else
  emi_425 : Assertion

== system sampleModel7293_pp_1_1_mu/cfblk205/cfblk5 ==
  emi_1043 : Inport
  Action Port : ActionPort  ActionType=then
  cfblk5 : DiscreteZeroPole  Poles=[0 0.5]  Gain=1  SampleTime=-1
  emi_1044 : Outport
  wires:
  emi_1043/1 -> cfblk5/1
  cfblk5/1 -> emi_1044/1

== system sampleModel7293_pp_1_1_mu/cfblk205/cfblk7 ==
  emi_2090 : Inport
  emi_2091 : Inport  Port=2
  Action Port : ActionPort  ActionType=then
  cfblk7 : simulink/Continuous/PID Controller (2DOF)  Controller=PID  TimeDomain=Discrete-time  SampleTime=-1  IntegratorMethod=Forward Euler  FilterMethod=Forward Euler  Form=Parallel  UseFilter=on  ControllerParametersSource=internal  P=1  I=1  D=0  N=100  b=1  c=1  InitialConditionSource=internal  InitialConditionForIntegrator=0  InitialConditionForFilter=0  ExternalReset=none  LimitOutput=off  UpperSaturationLimit=inf  LowerSaturationLimit=-inf  LinearizeAsGain=off  AntiWindupMode=none  Kb=1  TrackingMode=off  Kt=1  PParamMin=[]  PParamMax=[]  IParamMin=[]  IParamMax=[]  DParamMin=[]  DParamMax=[]  NParamMin=[]  NParamMax=[]  bParamMin=[]  bParamMax=[]  cParamMin=[]  cParamMax=[]  KbParamMin=[]  KbParamMax=[]  KtParamMin=[]  KtParamMax=[]  POutMin=[]  POutMax=[]  IOutMin=[]  IOutMax=[]  DOutMin=[]  DOutMax=[]  NOutMin=[]  NOutMax=[]  bOutMin=[]  bOutMax=[]  cOutMin=[]  cOutMax=[]  KbOutMin=[]  KbOutMax=[]  KtOutMin=[]  KtOutMax=[]  IntegratorOutMin=[]  IntegratorOutMax=[]  FilterOutMin=[]  FilterOutMax=[]  SumOutMin=[]  SumOutMax=[]  Sum1OutMin=[]  Sum1OutMax=[]  Sum2OutMin=[]  Sum2OutMax=[]  Sum3OutMin=[]  Sum3OutMax=[]  SumI1OutMin=[]  SumI1OutMax=[]  SumI2OutMin=[]  SumI2OutMax=[]  SumI3OutMin=[]  SumI3OutMax=[]  SumDOutMin=[]  SumDOutMax=[]  SaturationOutMin=[]  SaturationOutMax=[]  IntegratorContinuousStateAttributes=''  IntegratorStateMustResolveToSignalObject=off  IntegratorRTWStateStorageClass=Auto  FilterContinuousStateAttributes=''  FilterStateMustResolveToSignalObject=off  FilterRTWStateStorageClass=Auto  DifferentiatorICPrevScaledInput=0  DifferentiatorOutMin=[]  DifferentiatorOutMax=[]  FilterDiffOutCoefMin=[]  FilterDiffOutCoefMax=[]  SumDenOutMin=[]  SumDenOutMax=[]  SumNumOutMin=[]  SumNumOutMax=[]  ReciprocalOutMin=[]  ReciprocalOutMax=[]  DivideOutMin=[]  DivideOutMax=[]  TunerSelectOption=Transfer Function Based (PID Tuner App)
  emi_2092 : Outport
  wires:
  emi_2090/1 -> cfblk7/1
  emi_2091/1 -> cfblk7/2
  cfblk7/1 -> emi_2092/1

== system sampleModel7293_pp_1_1_mu/cfblk205/emi_1045 ==
  Action Port : ActionPort  ActionType=else
  emi_1046 : Assertion

== system sampleModel7293_pp_1_1_mu/cfblk205/emi_2093 ==
  Action Port : ActionPort  ActionType=else
  emi_2094 : Assertion

== system sampleModel7293_pp_1_1_mu/cfblk206/cfblk16 ==
  cfblk1 : Inport
  cfblk12 : Inport  Port=2
  Action Port : ActionPort  ActionType=then
  cfblk10 : simulink/Discrete/Difference  ICPrevInput=0.0  OutMin=[]  OutMax=[]  OutDataTypeStr=double  OutputDataTypeScalingMode=double  OutDataType=fixdt(1, 16)  OutScaling=2^-10  DoSatur=off
  cfblk11 : DiscreteFilter
  cfblk15 : Delay
  cfblk3 : Subsystem  TreatAsAtomicUnit=on
  cfblk4 : DiscreteIntegrator  SampleTime=-1  OutDataTypeStr=double  ICPrevOutput=DiscIntNeverNeededParam  ICPrevScaledInput=DiscIntNeverNeededParam
  cfblk5 : simulink/Continuous/PID Controller  Controller=PID  TimeDomain=Discrete-time  SampleTime=-1  IntegratorMethod=Forward Euler  FilterMethod=Forward Euler  Form=Parallel  UseFilter=on  ControllerParametersSource=internal  P=1  I=1  D=0  N=100  InitialConditionSource=internal  InitialConditionForIntegrator=0  InitialConditionForFilter=0  ExternalReset=none  LimitOutput=off  UpperSaturationLimit=inf  LowerSaturationLimit=-inf  LinearizeAsGain=off  AntiWindupMode=none  Kb=1  TrackingMode=off  Kt=1  PParamMin=[]  PParamMax=[]  IParamMin=[]  IParamMax=[]  DParamMin=[]  DParamMax=[]  NParamMin=[]  NParamMax=[]  KbParamMin=[]  KbParamMax=[]  KtParamMin=[]  KtParamMax=[]  POutMin=[]  POutMax=[]  IOutMin=[]  IOutMax=[]  DOutMin=[]  DOutMax=[]  NOutMin=[]  NOutMax=[]  KbOutMin=[]  KbOutMax=[]  KtOutMin=[]  KtOutMax=[]  IntegratorOutMin=[]  IntegratorOutMax=[]  FilterOutMin=[]  FilterOutMax=[]  SumOutMin=[]  SumOutMax=[]  SumI1OutMin=[]  SumI1OutMax=[]  SumI2OutMin=[]  SumI2OutMax=[]  SumI3OutMin=[]  SumI3OutMax=[]  SumDOutMin=[]  SumDOutMax=[]  SaturationOutMin=[]  SaturationOutMax=[]  IntegratorContinuousStateAttributes=''  IntegratorStateMustResolveToSignalObject=off  IntegratorRTWStateStorageClass=Auto  FilterContinuousStateAttributes=''  FilterStateMustResolveToSignalObject=off  FilterRTWStateStorageClass=Auto  DifferentiatorICPrevScaledInput=0  DifferentiatorOutMin=[]  DifferentiatorOutMax=[]  FilterDiffOutCoefMin=[]  FilterDiffOutCoefMax=[]  SumDenOutMin=[]  SumDenOutMax=[]  SumNumOutMin=[]  SumNumOutMax=[]  ReciprocalOutMin=[]  ReciprocalOutMax=[]  DivideOutMin=[]  DivideOutMax=[]  TunerSelectOption=Transfer Function Based (PID Tuner App)
  cfblk6 : Subsystem  TreatAsAtomicUnit=on
  cfblk7 : Delay
  cfblk8 : Subsystem  TreatAsAtomicUnit=on
  cfblk9 : UnitDelay  SampleTime=-1
  cyemi_{1278..1287} (10 alike) : DataTypeConversion  OutDataTypeStr=double
  emi_1624 : Subsystem  TreatAsAtomicUnit=on
  emi_1626 : If  IfExpression=Inf <= u1
  emi_1627 : DataTypeConversion  OutDataTypeStr=double
  emi_1795 : Subsystem  TreatAsAtomicUnit=on
  emi_1797 : If  IfExpression=Inf <= u1
  emi_1798 : DataTypeConversion  OutDataTypeStr=double
  emi_2114 : Subsystem  TreatAsAtomicUnit=on
  emi_2116 : If  IfExpression=Inf <= u1
  emi_2117 : DataTypeConversion  OutDataTypeStr=double
  cfblk2 : Outport
  cfblk13 : Outport  Port=2
  cfblk14 : Outport  Port=3
  wires:
  cfblk10/1 -> cfblk14/1
  cfblk5/1 -> cfblk2/1, cyemi_1284/1
  cyemi_1278/1 -> cfblk10/1
  cfblk4/1 -> cyemi_1278/1, emi_1798/1, emi_2117/1
  cyemi_1279/1 -> cfblk11/1
  cfblk1/1 -> cyemi_1279/1
  cyemi_1280/1 -> cfblk15/1
  cfblk12/1 -> cyemi_1281/1
  cyemi_1282/1 -> cfblk4/1
  cfblk7/1 -> cyemi_1282/1
  cyemi_1283/1 -> cfblk5/1
  cfblk15/1 -> cyemi_1283/1
  cyemi_1285/1 -> cfblk7/1
  cfblk9/1 -> cyemi_1285/1
  cyemi_1287/1 -> cfblk9/1
  cfblk11/1 -> cyemi_1287/1, emi_1627/1
  cyemi_1281/1 -> cfblk3/1(emi_1622)
  cfblk3/1(emi_1623) -> cfblk13/1
  emi_1626/1 -> cfblk3/Action
  emi_1626/2 -> emi_1624/Action
  emi_1627/1 -> emi_1626/1
  cyemi_1284/1 -> cfblk6/1(emi_1793)
  cfblk6/1(emi_1794) -> cyemi_1286/1
  emi_1797/1 -> cfblk6/Action
  emi_1797/2 -> emi_1795/Action
  emi_1798/1 -> emi_1797/1
  cyemi_1286/1 -> cfblk8/1(emi_2112)
  cfblk8/1(emi_2113) -> cyemi_1280/1
  emi_2116/1 -> cfblk8/Action
  emi_2116/2 -> emi_2114/Action
  emi_2117/1 -> emi_2116/1

== system sampleModel7293_pp_1_1_mu/cfblk206/cfblk17 ==
  cfblk1 : Inport
  cfblk7 : Inport  Port=2
  Action Port : ActionPort  ActionType=else
  cfblk3 : DiscreteZeroPole  Poles=[0 0.5]  Gain=1  SampleTime=-1
  cfblk4 : Subsystem  TreatAsAtomicUnit=on
  cfblk5 : DiscreteFilter
  cfblk6 : DiscreteStateSpace  SampleTime=-1
  cfblk8 : Delay
  cyemi_{1290..1294} (5 alike) : DataTypeConversion  OutDataTypeStr=double
  emi_1438 : Subsystem  TreatAsAtomicUnit=on
  emi_1440 : If  IfExpression=Inf <= u1
  emi_1441 : DataTypeConversion  OutDataTypeStr=double
  cfblk2 : Outport
  wires:
  cfblk3/1 -> cfblk2/1
  cyemi_1290/1 -> cfblk3/1
  cfblk1/1 -> cyemi_1291/1
  cyemi_1292/1 -> cfblk5/1
  cfblk8/1 -> cyemi_1292/1
  cyemi_1293/1 -> cfblk6/1
  cfblk5/1 -> cyemi_1293/1
  cyemi_1294/1 -> cfblk8/1
  cfblk6/1 -> cyemi_1294/1, emi_1441/1
  cyemi_1291/1 -> cfblk4/1(emi_1436)
  cfblk4/1(emi_1437) -> cyemi_1290/1
  emi_1440/1 -> cfblk4/Action
  emi_1440/2 -> emi_1438/Action
  emi_1441/1 -> emi_1440/1

== system sampleModel7293_pp_1_1_mu/cfblk206/cfblk19 ==
  emi_2033 : Inport
  Action Port : ActionPort  ActionType=then
  cfblk19 : Delay
  emi_2034 : Outport
  wires:
  emi_2033/1 -> cfblk19/1
  cfblk19/1 -> emi_2034/1

== system sampleModel7293_pp_1_1_mu/cfblk206/emi_2035 ==
  Action Port : ActionPort  ActionType=else
  emi_2036 : Assertion

== system sampleModel7293_pp_1_1_mu/cfblk208/cfblk15 ==
  emi_1934 : Inport
  Action Port : ActionPort  ActionType=then
  cfblk15 : Delay
  emi_1935 : Outport
  wires:
  emi_1934/1 -> cfblk15/1
  cfblk15/1 -> emi_1935/1

== system sampleModel7293_pp_1_1_mu/cfblk208/cfblk6 ==
  emi_1050 : Inport
  Action Port : ActionPort  ActionType=then
  cfblk6 : DiscreteStateSpace  SampleTime=-1
  emi_1051 : Outport
  wires:
  emi_1050/1 -> cfblk6/1
  cfblk6/1 -> emi_1051/1

== system sampleModel7293_pp_1_1_mu/cfblk208/cfblk7 ==
  emi_1564 : Inport
  Action Port : ActionPort  ActionType=then
  cfblk7 : simulink/Discrete/Transfer Fcn Lead or Lag  PoleZ=0.95  ZeroZ=0.75  ICPrevOutput=0.0  ICPrevInput=0.0  DoSatur=off
      settings: SourceProductName=Simulink  SourceProductBaseCode=SL
  emi_1565 : Outport
  wires:
  emi_1564/1 -> cfblk7/1
  cfblk7/1 -> emi_1565/1

== system sampleModel7293_pp_1_1_mu/cfblk208/cfblk9 ==
  emi_624 : Inport
  emi_625 : Inport  Port=2
  Action Port : ActionPort  ActionType=then
  cfblk9 : Delay  DelayLengthSource=Input port
      settings: InputPortMap=u0,p1
  emi_626 : Outport
  wires:
  emi_624/1 -> cfblk9/1
  emi_625/1 -> cfblk9/2
  cfblk9/1 -> emi_626/1

== system sampleModel7293_pp_1_1_mu/cfblk208/emi_1052 ==
  Action Port : ActionPort  ActionType=else
  emi_1053 : Assertion

== system sampleModel7293_pp_1_1_mu/cfblk208/emi_1566 ==
  Action Port : ActionPort  ActionType=else
  emi_1567 : Assertion

== system sampleModel7293_pp_1_1_mu/cfblk208/emi_1936 ==
  Action Port : ActionPort  ActionType=else
  emi_1937 : Assertion

== system sampleModel7293_pp_1_1_mu/cfblk208/emi_627 ==
  Action Port : ActionPort  ActionType=else
  emi_628 : Assertion

== system sampleModel7293_pp_1_1_mu/cfblk209/cfblk10 ==
  cfblk1 : Inport
  cfblk12 : Inport  Port=2
  Action Port : ActionPort  ActionType=else
  cfblk10 : DiscreteZeroPole  Poles=[0 0.5]  Gain=1  SampleTime=-1
  cfblk11 : Subsystem  TreatAsAtomicUnit=on
  cfblk15 : Delay
  cfblk3 : simulink/Discrete/Transfer Fcn Lead or Lag  PoleZ=0.95  ZeroZ=0.75  ICPrevOutput=0.0  ICPrevInput=0.0  DoSatur=off
      settings: SourceProductName=Simulink  SourceProductBaseCode=SL
  cfblk4 : simulink/Continuous/PID Controller  Controller=PID  TimeDomain=Discrete-time  SampleTime=-1  IntegratorMethod=Forward Euler  FilterMethod=Forward Euler  Form=Parallel  UseFilter=on  ControllerParametersSource=internal  P=1  I=1  D=0  N=100  InitialConditionSource=internal  InitialConditionForIntegrator=0  InitialConditionForFilter=0  ExternalReset=none  LimitOutput=off  UpperSaturationLimit=inf  LowerSaturationLimit=-inf  LinearizeAsGain=off  AntiWindupMode=none  Kb=1  TrackingMode=off  Kt=1  PParamMin=[]  PParamMax=[]  IParamMin=[]  IParamMax=[]  DParamMin=[]  DParamMax=[]  NParamMin=[]  NParamMax=[]  KbParamMin=[]  KbParamMax=[]  KtParamMin=[]  KtParamMax=[]  POutMin=[]  POutMax=[]  IOutMin=[]  IOutMax=[]  DOutMin=[]  DOutMax=[]  NOutMin=[]  NOutMax=[]  KbOutMin=[]  KbOutMax=[]  KtOutMin=[]  KtOutMax=[]  IntegratorOutMin=[]  IntegratorOutMax=[]  FilterOutMin=[]  FilterOutMax=[]  SumOutMin=[]  SumOutMax=[]  SumI1OutMin=[]  SumI1OutMax=[]  SumI2OutMin=[]  SumI2OutMax=[]  SumI3OutMin=[]  SumI3OutMax=[]  SumDOutMin=[]  SumDOutMax=[]  SaturationOutMin=[]  SaturationOutMax=[]  IntegratorContinuousStateAttributes=''  IntegratorStateMustResolveToSignalObject=off  IntegratorRTWStateStorageClass=Auto  FilterContinuousStateAttributes=''  FilterStateMustResolveToSignalObject=off  FilterRTWStateStorageClass=Auto  DifferentiatorICPrevScaledInput=0  DifferentiatorOutMin=[]  DifferentiatorOutMax=[]  FilterDiffOutCoefMin=[]  FilterDiffOutCoefMax=[]  SumDenOutMin=[]  SumDenOutMax=[]  SumNumOutMin=[]  SumNumOutMax=[]  ReciprocalOutMin=[]  ReciprocalOutMax=[]  DivideOutMin=[]  DivideOutMax=[]  TunerSelectOption=Transfer Function Based (PID Tuner App)
  cfblk5 : DiscreteIntegrator  SampleTime=-1  OutDataTypeStr=double  ICPrevOutput=DiscIntNeverNeededParam  ICPrevScaledInput=DiscIntNeverNeededParam
  cfblk6 : DiscreteFilter
  cfblk7 : Delay  DelayLengthSource=Input port
      settings: InputPortMap=u0,p1
  cfblk8 : simulink/Discrete/Transfer Fcn Real Zero  ZeroZ=0.75  ICPrevInput=0.0  DoSatur=off
      settings: SourceProductName=Simulink  SourceProductBaseCode=SL
  cfblk9 : UnitDelay  SampleTime=-1
  cyemi_{1330..1340} (11 alike) : DataTypeConversion  OutDataTypeStr=double
  emi_3 : Subsystem  TreatAsAtomicUnit=on
  emi_5 : If  IfExpression=0 <= u1
  emi_6 : DataTypeConversion  OutDataTypeStr=double
  cfblk2 : Outport
  cfblk13 : Outport  Port=2
  cfblk14 : Outport  Port=3
  wires:
  cfblk8/1 -> cfblk13/1, cyemi_1332/1
  cfblk1/1 -> cfblk2/1
  cfblk4/1 -> cfblk14/1, cyemi_1338/1
  cyemi_1330/1 -> cfblk10/1
  cfblk12/1 -> cyemi_1331/1
  cyemi_1332/1 -> cfblk15/1
  cyemi_1333/1 -> cfblk3/1
  cfblk15/1 -> cyemi_1333/1
  cyemi_1334/1 -> cfblk4/1
  cfblk3/1 -> cyemi_1334/1
  cyemi_1335/1 -> cfblk5/1
  cfblk6/1 -> cyemi_1335/1
  cyemi_1336/1 -> cfblk6/1
  cfblk7/1 -> cyemi_1336/1
  cyemi_1337/1 -> cfblk7/1
  cfblk10/1 -> cyemi_1337/1, emi_6/1
  cyemi_1338/1 -> cfblk7/2
  cyemi_1339/1 -> cfblk8/1
  cfblk9/1 -> cyemi_1339/1
  cyemi_1340/1 -> cfblk9/1
  cfblk5/1 -> cyemi_1340/1
  cyemi_1331/1 -> cfblk11/1(emi_1)
  cfblk11/1(emi_2) -> cyemi_1330/1
  emi_5/1 -> cfblk11/Action
  emi_5/2 -> emi_3/Action
  emi_6/1 -> emi_5/1

== system sampleModel7293_pp_1_1_mu/cfblk209/cfblk12 ==
  emi_1906 : Inport
  Action Port : ActionPort  ActionType=then
  cfblk12 : Delay
  emi_1907 : Outport
  wires:
  emi_1906/1 -> cfblk12/1
  cfblk12/1 -> emi_1907/1

== system sampleModel7293_pp_1_1_mu/cfblk209/cfblk4 ==
  emi_781 : Inport
  Action Port : ActionPort  ActionType=then
  cfblk4 : DiscreteFir
  emi_782 : Outport
  wires:
  emi_781/1 -> cfblk4/1
  cfblk4/1 -> emi_782/1

== system sampleModel7293_pp_1_1_mu/cfblk209/cfblk6 ==
  emi_1700 : Inport
  Action Port : ActionPort  ActionType=then
  cfblk6 : simulink/Discrete/Transfer Fcn Lead or Lag  PoleZ=0.95  ZeroZ=0.75  ICPrevOutput=0.0  ICPrevInput=0.0  DoSatur=off
      settings: SourceProductName=Simulink  SourceProductBaseCode=SL
  emi_1701 : Outport
  wires:
  emi_1700/1 -> cfblk6/1
  cfblk6/1 -> emi_1701/1
